simulink model "S120_smit"  (Simulink 8.9)
settings: Solver=VariableStepAuto  StartTime=0.0  StopTime=.1  FixedStep=.0000020833  RelTol=1e-6
undefined symbols (not defined in the file): T, T10, T20, T30, T40, T50, T60
settings Model: SuppressorTable=22 serialization::archive 11 0 6 0 0 0 0 0  Creator=1  LastModifiedBy=iusupova
settings DataIOCC: LimitDataPoints=off  SaveFormat=Dataset  SignalLoggingSaveFormat=Dataset
settings OptimizationCC: LifeSpan=auto
settings DebuggingCC: UnderspecifiedInitializationDetection=Simplified  MergeDetectMultiDrivingBlocksExec=error  FcnCallInpInsideContextMsg=error  StateNameClashWarn=none  SFUnexpectedBacktrackingDiag=error  SFNoUnconditionalDefaultTransitionDiag=error  SFExecutionAtInitializationDiag=warning
settings HardwareCC: ProdBitPerPointer=64  ProdBitPerSizeT=64  ProdBitPerPtrDiffT=64  ProdLargestAtomicFloat=Float  ProdIntDivRoundTo=Zero  ProdEndianess=LittleEndian  ProdWordSize=64  ProdHWDeviceType=Intel->x86-64 (Windows64)
settings ModelReferenceCC: PropagateSignalLabelsOutOfModel=on
settings GRTTargetCC: TargetLangStandard=C99 (ISO)  GeneratePreprocessorConditionals=Use local settings  CombineOutputUpdateFcns=on  GRTInterface=off
settings ConfigComp: CovMetricSettings=dwe  CovHtmlReporting=off  CovSaveCumulativeToWorkspaceVar=off  CovSaveSingleToWorkspaceVar=off  CovExternalEMLEnable=on

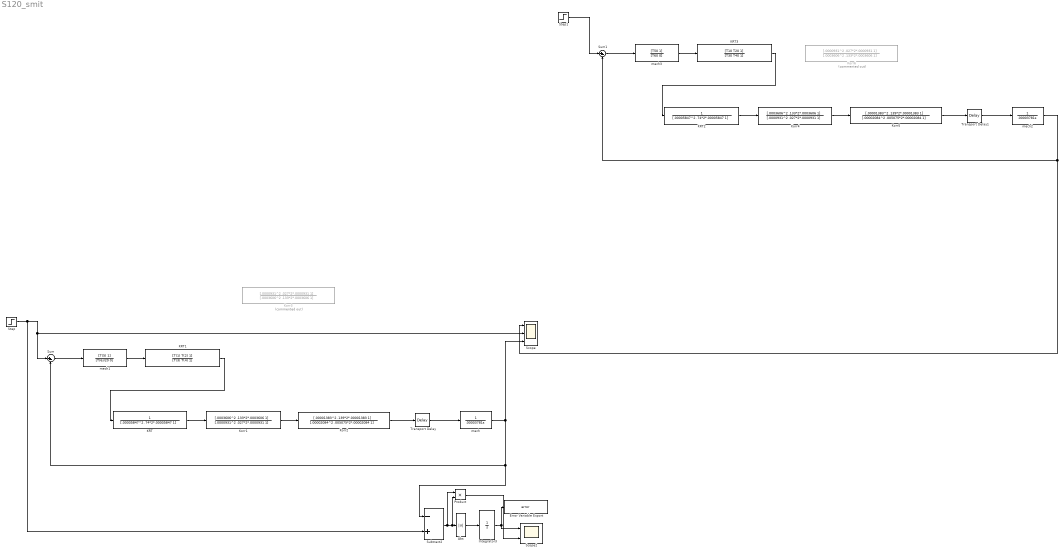
== system S120_smit ==
  Abs : Abs
  Error Variable Export : ToWorkspace  VariableName=error  SampleTime=-1
      settings: Save2DSignal=2-D array (concatenate along first dimension)
  Integrator3 : Integrator  IgnoreLimit=on
  KRT : TransferFcn  Denominator=[.00005847^2 .74*2*.00005847 1]
  KRT1 : TransferFcn  Numerator=[T(1) T(2) 1]  Denominator=[T(3) T(4) 1]
  KRT2 : TransferFcn  Denominator=[.00005847^2 .74*2*.00005847 1]
  KRT3 : TransferFcn  Numerator=[T10 T20 1]  Denominator=[T30 T40 1]
  Korr1 : TransferFcn  Numerator=[.0003606^2 .133*2*.0003606 1]  Denominator=[.0000931^2 .027*2*.0000931 1]
  Korr2 : TransferFcn  Numerator=[.00001383^2 .139*2*.00001383 1]  Denominator=[.00002084^2 .005075*2*.00002084 1]
  Korr3 : TransferFcn  Commented=on  Numerator=[.0000931^2 .027*2*.0000931 1]  Denominator=[.0003606^2 .133*2*.0003606 1]
  Korr4 : TransferFcn  Numerator=[.0003606^2 .133*2*.0003606 1]  Denominator=[.0000931^2 .027*2*.0000931 1]
  Korr5 : TransferFcn  Numerator=[.00001383^2 .139*2*.00001383 1]  Denominator=[.00002084^2 .005075*2*.00002084 1]
  Korr6 : TransferFcn  Commented=on  Numerator=[.0000931^2 .027*2*.0000931 1]  Denominator=[.0003606^2 .133*2*.0003606 1]
  Product : Product
  Scope : Scope  NumInputPorts=3
  Scope2 : Scope  NumInputPorts=2
  Step : Step  Time=.001  SampleTime=0
  Step1 : Step  Time=.001  SampleTime=0
  Subtract2 : Sum  Inputs=-+
  Sum : Sum  Inputs=|+-
  Sum1 : Sum  Inputs=|+-
  Transport Delay : TransportDelay  DelayTime=.0001424
  Transport Delay1 : TransportDelay  DelayTime=.0001424
  mech : TransferFcn  Denominator=[.00003781 0]
  mech1 : TransferFcn  Numerator=[T(5) 1]  Denominator=[T(6)/20 0]
  mech2 : TransferFcn  Denominator=[.00003781 0]
  mech3 : TransferFcn  Numerator=[T50 1]  Denominator=[T60 0]
  wires:
  Sum/1 -> mech1/1
  mech/1 -> Subtract2/1, Sum/2, Scope/3
  Step/1 -> Subtract2/2, Sum/1, Scope/2
  Integrator3/1 -> Error Variable Export/1, Scope2/1
  Subtract2/1 -> Product/2, Abs/1, Product/1
  Abs/1 -> Integrator3/1
  mech1/1 -> KRT1/1
  Transport Delay/1 -> mech/1
  Korr2/1 -> Transport Delay/1
  KRT1/1 -> KRT/1
  Korr1/1 -> Korr2/1
  KRT/1 -> Korr1/1
  Transport Delay1/1 -> mech2/1
  mech2/1 -> Scope/1, Sum1/2
  Korr5/1 -> Transport Delay1/1
  KRT3/1 -> KRT2/1
  Korr4/1 -> Korr5/1
  mech3/1 -> KRT3/1
  Sum1/1 -> mech3/1
  Step1/1 -> Sum1/1
  KRT2/1 -> Korr4/1
  Product/1 -> Scope2/2
